simulink model "halfwave_rectifierdigital15"  (R2024a)
settings: Solver=VariableStepAuto  StartTime=0.0  StopTime=10  RelTol=1e-3
libraries: simulink x3
settings Model: Creator=vijit  LastModifiedBy=tusha
settings OptimizationCC: ReuseModelBlockBuffer=off
settings RTWCC: GPUComputeCapability=3.5

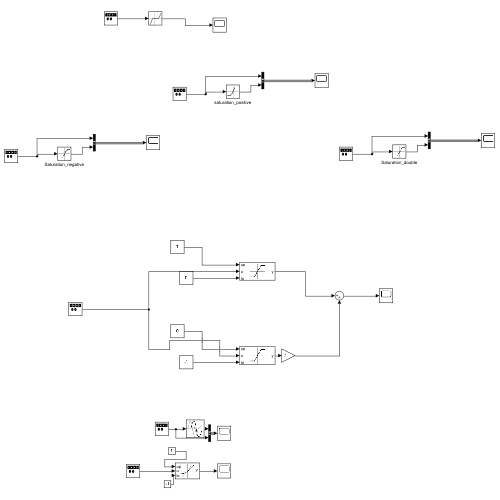
[thumbnail: Simulink's stored preview of the top-level diagram]
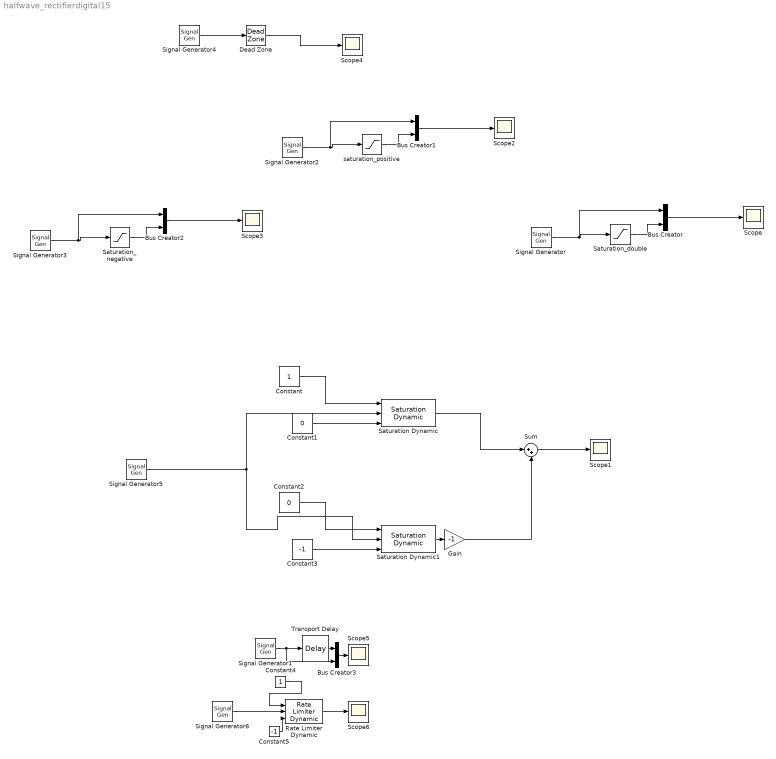
== system halfwave_rectifierdigital15 ==
  Bus Creator{,1..3} (4 alike) : BusCreator  Inputs=2
  Constant : Constant
  Constant1 : Constant  Value=0
  Constant2 : Constant  Value=0
  Constant3 : Constant  Value=-1
  Constant4 : Constant
  Constant5 : Constant  Value=-1
  Dead Zone : DeadZone  LowerValue=-0.25  UpperValue=0.25
  Gain : Gain  Gain=-1
  Rate Limiter Dynamic : simulink/Discontinuities/Rate Limiter Dynamic
  Saturation Dynamic : simulink/Discontinuities/Saturation Dynamic  OutMin=[]  OutMax=[]  OutDataTypeStr=Inherit: Same as second input  OutDataType=fixdt(1, 16)  OutScaling=2^-10  DoSatur=off
  Saturation Dynamic1 : simulink/Discontinuities/Saturation Dynamic  OutMin=[]  OutMax=[]  OutDataTypeStr=Inherit: Same as second input  OutDataType=fixdt(1, 16)  OutScaling=2^-10  DoSatur=off
  Saturation_double : Saturate
  Saturation_negative : Saturate  UpperLimit=1
  Scope{,1..6} (7 alike) : Scope
  Signal Generator{,1..3,5..6} (6 alike) : SignalGenerator  Units=rad/sec
  Signal Generator4 : SignalGenerator  Frequency=0.2  Units=rad/sec
  Sum : Sum  Inputs=|++
  Transport Delay : TransportDelay
  saturation_positive : Saturate  LowerLimit=-1
  wires:
  Constant1/1 -> Saturation Dynamic/3
  Constant/1 -> Saturation Dynamic/1
  Saturation_double/1 -> Bus Creator/2
  Signal Generator/1 -> Bus Creator/1, Saturation_double/1
  Bus Creator/1 -> Scope/1
  Signal Generator5/1 -> Saturation Dynamic1/2, Saturation Dynamic/2
  Saturation Dynamic/1 -> Sum/1
  Bus Creator1/1 -> Scope2/1
  saturation_positive/1 -> Bus Creator1/2
  Signal Generator2/1 -> Bus Creator1/1, saturation_positive/1
  Saturation_negative/1 -> Bus Creator2/2
  Bus Creator2/1 -> Scope3/1
  Signal Generator3/1 -> Bus Creator2/1, Saturation_negative/1
  Signal Generator4/1 -> Dead Zone/1
  Dead Zone/1 -> Scope4/1
  Constant2/1 -> Saturation Dynamic1/1
  Constant3/1 -> Saturation Dynamic1/3
  Saturation Dynamic1/1 -> Gain/1
  Gain/1 -> Sum/2
  Sum/1 -> Scope1/1
  Transport Delay/1 -> Bus Creator3/1
  Bus Creator3/1 -> Scope5/1
  Signal Generator1/1 -> Bus Creator3/2, Transport Delay/1
  Rate Limiter Dynamic/1 -> Scope6/1
  Signal Generator6/1 -> Rate Limiter Dynamic/2
  Constant4/1 -> Rate Limiter Dynamic/1
  Constant5/1 -> Rate Limiter Dynamic/3
